simulink model "Mis1"  (R2022b)
settings: Solver=VariableStepAuto  StartTime=0.0  StopTime=10000  MaxStep=1  RelTol=1e-3
undefined symbols (not defined in the file or in its folder): cpp, Cvp, Cvw, dPg0, dTzew0, Fp0, K1, Kd, Kp, Pg0, rop, t_skok, Tp0, Twew0, Tzew0
settings Model: Creator=matkw  LastModifiedBy=matkw

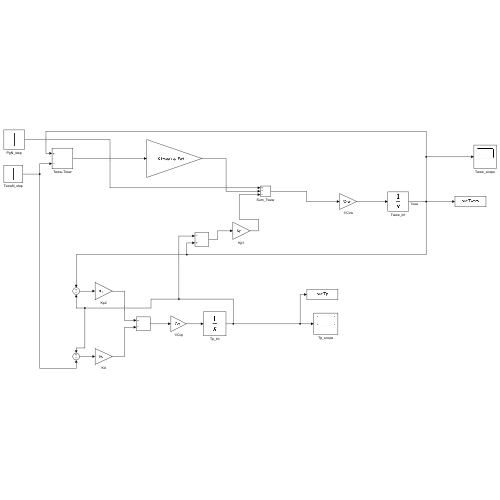
[thumbnail: Simulink's stored preview of the top-level diagram]
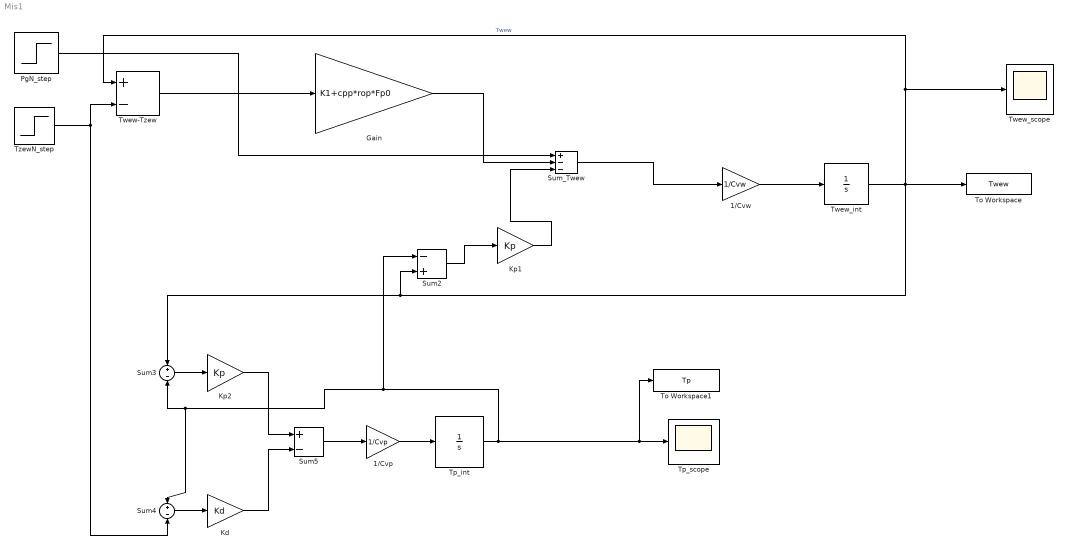
== system Mis1 ==
  1/Cvp : Gain  Gain=1/Cvp
  1/Cvw : Gain  Gain=1/Cvw
  Gain : Gain  Gain=K1+cpp*rop*Fp0
  Kd : Gain  Gain=Kd
  Kp1 : Gain  Gain=Kp
  Kp2 : Gain  Gain=Kp
  PgN_step : Step  Time=t_skok  Before=Pg0  After=Pg0+dPg0  SampleTime=0
  Sum2 : Sum  Inputs=-+
  Sum3 : Sum  Inputs=+-
  Sum4 : Sum  Inputs=+-
  Sum5 : Sum  Inputs=+-
  Sum_Twew : Sum  Inputs=+--
  To Workspace : ToWorkspace  VariableName=Twew  SampleTime=-1
  To Workspace1 : ToWorkspace  VariableName=Tp  SampleTime=-1
  Tp_int : Integrator  InitialCondition=Tp0
  Tp_scope : Scope
  Twew-Tzew : Sum  Inputs=+-
  Twew_int : Integrator  InitialCondition=Twew0
  Twew_scope : Scope
  TzewN_step : Step  Time=t_skok  Before=Tzew0  After=Tzew0+dTzew0  SampleTime=1000
  wires:
  Twew_int/1 -> To Workspace/1, Twew-Tzew/1, Twew_scope/1, Sum3/1, Sum2/2  "Twew"
  TzewN_step/1 -> Sum4/2, Twew-Tzew/2
  Twew-Tzew/1 -> Gain/1
  Sum2/1 -> Kp1/1
  Sum_Twew/1 -> 1/Cvw/1
  1/Cvw/1 -> Twew_int/1
  Sum3/1 -> Kp2/1
  Sum4/1 -> Kd/1
  Kp2/1 -> Sum5/1
  Kd/1 -> Sum5/2
  Sum5/1 -> 1/Cvp/1
  1/Cvp/1 -> Tp_int/1
  Tp_int/1 -> Sum2/1, Sum3/2, Sum4/1, To Workspace1/1, Tp_scope/1
  Kp1/1 -> Sum_Twew/3
  Gain/1 -> Sum_Twew/2
  PgN_step/1 -> Sum_Twew/1
